simulink model "motor_model"  (R2022a)
settings: Solver=VariableStepAuto  StartTime=0.0  StopTime=T  FixedStep=0.001  RelTol=1e-3
values from neighbouring files (symbols this model uses):
  den_sys = sys.den{:}    [main.m]
  Kd = 10    [main.m]
  Ki = 100    [main.m]
  Kp = 300    [main.m]
  N = 80    [main.m]
  num_sys = sys.num{:}    [main.m]
undefined symbols (not defined in the file or in its folder): C_csd_den, C_csd_num, den_si, num_si
libraries: slpidlib x2, simulink x1
settings Model: Creator=michi  LastModifiedBy=michi

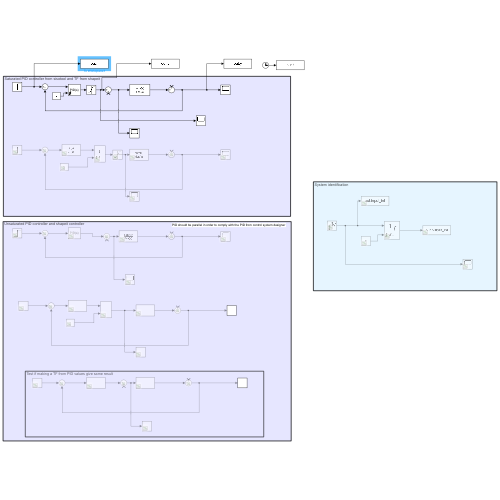
[thumbnail: Simulink's stored preview of the top-level diagram]
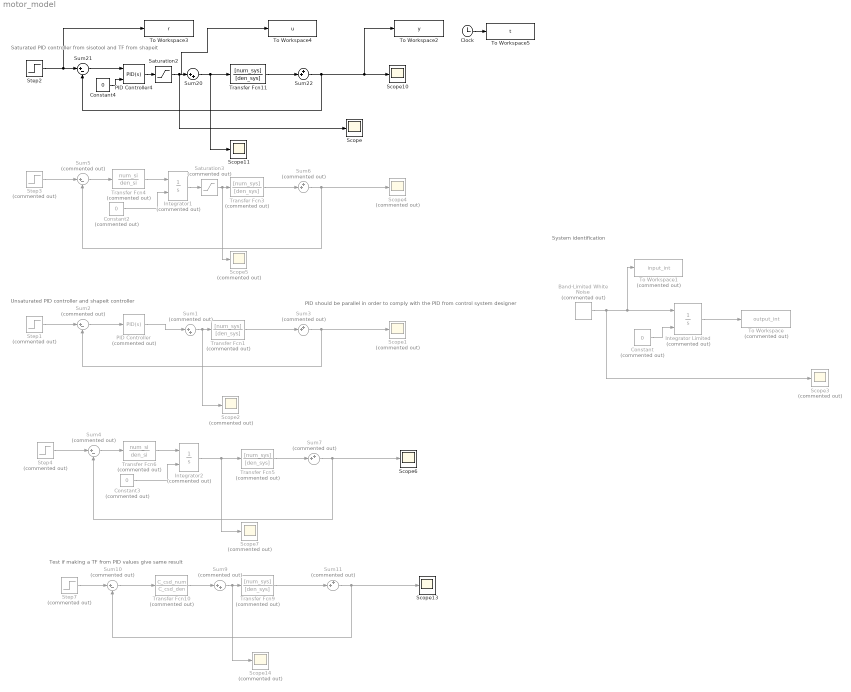
== system motor_model ==
  note: Test if making a TF from PID values give same result
  note: System identification
  note: PID should be parallel in order to comply with the PID from control system designer
  note: Unsaturated PID controller and shapeit controller
  note: Saturated PID controller from sisotool and TF from shapeit
  Band-Limited White Noise : simulink/Sources/Band-Limited White Noise  Commented=on  Cov=[1]  Ts=0.001  seed=[23341]
  Clock : Clock
  Constant : Constant  Commented=on  Value=0
  Constant2 : Constant  Commented=on  Value=0
  Constant3 : Constant  Commented=on  Value=0
  Constant4 : Constant  Value=0
  Integrator Limited : Integrator  Commented=on  ExternalReset=rising  LimitOutput=on  UpperSaturationLimit=3  LowerSaturationLimit=-3
  Integrator1 : Integrator  Commented=on  ExternalReset=rising  UpperSaturationLimit=3  LowerSaturationLimit=-3
  Integrator2 : Integrator  Commented=on  ExternalReset=rising  UpperSaturationLimit=3  LowerSaturationLimit=-3
  PID Controller : slpidlib/PID Controller  Commented=on  Controller=PID  Form=Parallel  TimeDomain=Continuous-time  UseExternalTs=off  SampleTime=-1  IntegratorMethod=Forward Euler  FilterMethod=Forward Euler  ControllerParametersSource=internal  P=Kp  I=Ki  UseKiTs=off  D=Kd  N=N  UseFilter=on  TunerSelectOption=Transfer Function Based (PID Tuner App)  InitialConditionSource=internal  InitialConditionForIntegrator=0  InitialConditionForFilter=0  DifferentiatorICPrevScaledInput=0  ExternalReset=none  TrackingMode=off  Kt=1  LimitOutput=off  SatLimitsSource=internal  UpperSaturationLimit=inf  LowerSaturationLimit=-inf  LinearizeAsGain=on  AntiWindupMode=none  Kb=1  POutMin=[]  POutMax=[]  IOutMin=[]  IOutMax=[]  DOutMin=[]  DOutMax=[]  NOutMin=[]  NOutMax=[]  SumOutMin=[]  SumOutMax=[]  SaturationOutMin=[]  SaturationOutMax=[]  PParamMin=[]  PParamMax=[]  IParamMin=[]  IParamMax=[]  DParamMin=[]  DParamMax=[]  NParamMin=[]  NParamMax=[]  KbParamMin=[]  KbParamMax=[]  KtParamMin=[]  KtParamMax=[]  KbOutMin=[]  KbOutMax=[]  KtOutMin=[]  KtOutMax=[]  IntegratorOutMin=[]  IntegratorOutMax=[]  FilterOutMin=[]  FilterOutMax=[]  SumI1OutMin=[]  SumI1OutMax=[]  SumI2OutMin=[]  SumI2OutMax=[]  SumI3OutMin=[]  SumI3OutMax=[]  SumI4OutMin=[]  SumI4OutMax=[]  SumDOutMin=[]  SumDOutMax=[]  DifferentiatorOutMin=[]  DifferentiatorOutMax=[]  FilterDiffOutCoefMin=[]  FilterDiffOutCoefMax=[]  ReciprocalOutMin=[]  ReciprocalOutMax=[]  SumDenOutMin=[]  SumDenOutMax=[]  SumNumOutMin=[]  SumNumOutMax=[]  DivideOutMin=[]  DivideOutMax=[]  UdiffTsProdOutMin=[]  UdiffTsProdOutMax=[]  NTsProdOutMin=[]  NTsProdOutMax=[]  UintegralTsProdOutMin=[]  UintegralTsProdOutMax=[]  UngainTsProdOutMin=[]  UngainTsProdOutMax=[]  IntegratorContinuousStateAttributes=''  IntegratorStateMustResolveToSignalObject=off  IntegratorRTWStateStorageClass=Auto  FilterContinuousStateAttributes=''  FilterStateMustResolveToSignalObject=off  FilterRTWStateStorageClass=Auto  ParallelPVariant=InternalParameters  IdealPVariant=Disabled  IVariant=InternalParameters  DVariant=InternalParameters  IntegratorVariant=Continuous  SatVariant=Disabled  AWVariant=Passthrough  PCopyVariant=Disabled  TRVariant=Disabled  FdbkBlocksVariant=Forward  IdealPFdbkVariant=Disabled  SatFdbkVariant=Disabled  DerivativeFilterVariant=ContFilter  NVariant=InternalParameters  NCopyVariant=Disabled  FilterICVariant=InternalICsFilter  IntegratorICVariant=InternalICs  ExternalResetVariant=Disabled  TRSumVariant=Passthrough  SumFdbkVariant=Disabled  SumVariant=Sum_PID  TsampFilterVariant=InternalTs  TsampNgainVariant=Passthrough  TsampIntegralVariant=Passthrough  ExternalSaturationOutDataTypeStr=Inherit: Same as second input  aMode=0
  PID Controller4 : slpidlib/PID Controller  Controller=PID  Form=Parallel  TimeDomain=Continuous-time  UseExternalTs=off  SampleTime=-1  IntegratorMethod=Forward Euler  FilterMethod=Forward Euler  ControllerParametersSource=internal  P=Kp  I=Ki  UseKiTs=off  D=Kd  N=N  UseFilter=on  TunerSelectOption=Transfer Function Based (PID Tuner App)  InitialConditionSource=internal  InitialConditionForIntegrator=0  InitialConditionForFilter=0  DifferentiatorICPrevScaledInput=0  ExternalReset=rising  TrackingMode=off  Kt=1  LimitOutput=off  SatLimitsSource=internal  UpperSaturationLimit=inf  LowerSaturationLimit=-inf  LinearizeAsGain=on  AntiWindupMode=none  Kb=1  POutMin=[]  POutMax=[]  IOutMin=[]  IOutMax=[]  DOutMin=[]  DOutMax=[]  NOutMin=[]  NOutMax=[]  SumOutMin=[]  SumOutMax=[]  SaturationOutMin=[]  SaturationOutMax=[]  PParamMin=[]  PParamMax=[]  IParamMin=[]  IParamMax=[]  DParamMin=[]  DParamMax=[]  NParamMin=[]  NParamMax=[]  KbParamMin=[]  KbParamMax=[]  KtParamMin=[]  KtParamMax=[]  KbOutMin=[]  KbOutMax=[]  KtOutMin=[]  KtOutMax=[]  IntegratorOutMin=[]  IntegratorOutMax=[]  FilterOutMin=[]  FilterOutMax=[]  SumI1OutMin=[]  SumI1OutMax=[]  SumI2OutMin=[]  SumI2OutMax=[]  SumI3OutMin=[]  SumI3OutMax=[]  SumI4OutMin=[]  SumI4OutMax=[]  SumDOutMin=[]  SumDOutMax=[]  DifferentiatorOutMin=[]  DifferentiatorOutMax=[]  FilterDiffOutCoefMin=[]  FilterDiffOutCoefMax=[]  ReciprocalOutMin=[]  ReciprocalOutMax=[]  SumDenOutMin=[]  SumDenOutMax=[]  SumNumOutMin=[]  SumNumOutMax=[]  DivideOutMin=[]  DivideOutMax=[]  UdiffTsProdOutMin=[]  UdiffTsProdOutMax=[]  NTsProdOutMin=[]  NTsProdOutMax=[]  UintegralTsProdOutMin=[]  UintegralTsProdOutMax=[]  UngainTsProdOutMin=[]  UngainTsProdOutMax=[]  IntegratorContinuousStateAttributes=''  IntegratorStateMustResolveToSignalObject=off  IntegratorRTWStateStorageClass=Auto  FilterContinuousStateAttributes=''  FilterStateMustResolveToSignalObject=off  FilterRTWStateStorageClass=Auto  ParallelPVariant=InternalParameters  IdealPVariant=Disabled  IVariant=InternalParameters  DVariant=InternalParameters  IntegratorVariant=Continuous  SatVariant=Disabled  AWVariant=Passthrough  PCopyVariant=Disabled  TRVariant=Disabled  FdbkBlocksVariant=Forward  IdealPFdbkVariant=Disabled  SatFdbkVariant=Disabled  DerivativeFilterVariant=ContFilter  NVariant=InternalParameters  NCopyVariant=Disabled  FilterICVariant=InternalICsFilter  IntegratorICVariant=InternalICs  ExternalResetVariant=ExternalReset  TRSumVariant=Passthrough  SumFdbkVariant=Disabled  SumVariant=Sum_PID  TsampFilterVariant=InternalTs  TsampNgainVariant=Passthrough  TsampIntegralVariant=Passthrough  ExternalSaturationOutDataTypeStr=Inherit: Same as second input  aMode=0
  Saturation2 : Saturate  UpperLimit=3  LowerLimit=-3
  Saturation3 : Saturate  Commented=on  UpperLimit=3  LowerLimit=-3
  Scope{,6,10..11,13} (5 alike) : Scope
  Scope{1..5,7,14} (7 alike) : Scope  Commented=on
  Step{1,3..4,7} (4 alike) : Step  Commented=on  After=0.01  SampleTime=0
  Step2 : Step  Before=-0.02  After=0.02  SampleTime=0
  Sum1 : Sum  Commented=on  Inputs=|++
  Sum{2,4..5,10} (4 alike) : Sum  Commented=on  Inputs=|+-
  Sum{3,6..7,11} (4 alike) : Sum  Commented=on  Inputs=++|
  Sum20 : Sum  Inputs=|++
  Sum21 : Sum  Inputs=|+-
  Sum22 : Sum  Inputs=++|
  Sum9 : Sum  Commented=on  Inputs=|++
  To Workspace : ToWorkspace  Commented=on  VariableName=output_int  SampleTime=-1
  To Workspace1 : ToWorkspace  Commented=on  VariableName=input_int  SampleTime=-1
  To Workspace2 : ToWorkspace  VariableName=y  SampleTime=-1
  To Workspace3 : ToWorkspace  VariableName=r  SampleTime=-1
  To Workspace4 : ToWorkspace  VariableName=u  SampleTime=-1
  To Workspace5 : ToWorkspace  VariableName=t  SampleTime=-1
  Transfer Fcn{1,3,5,9} (4 alike) : TransferFcn  Commented=on  Numerator=[num_sys]  Denominator=[den_sys]
  Transfer Fcn10 : TransferFcn  Commented=on  Numerator=C_csd_num  Denominator=C_csd_den
  Transfer Fcn11 : TransferFcn  Numerator=[num_sys]  Denominator=[den_sys]
  Transfer Fcn4 : TransferFcn  Commented=on  Numerator=num_si  Denominator=den_si
  Transfer Fcn6 : TransferFcn  Commented=on  Numerator=num_si  Denominator=den_si
  wires:
  Constant/1 -> Integrator Limited/2
  Band-Limited White Noise/1 -> Scope3/1, To Workspace1/1, Integrator Limited/1
  Integrator Limited/1 -> To Workspace/1
  PID Controller4/1 -> Saturation2/1
  Sum21/1 -> PID Controller4/1
  Sum20/1 -> Transfer Fcn11/1, Scope11/1
  Constant4/1 -> PID Controller4/2
  Step2/1 -> To Workspace3/1, Sum21/1
  Saturation2/1 -> Scope/1, To Workspace4/1, Sum20/1
  Sum22/1 -> To Workspace2/1, Scope10/1, Sum21/2
  Sum3/1 -> Scope1/1, Sum2/2
  Transfer Fcn1/1 -> Sum3/2
  Step1/1 -> Sum2/1
  Sum1/1 -> Scope2/1, Transfer Fcn1/1
  Step3/1 -> Sum5/1
  Sum6/1 -> Scope4/1, Sum5/2
  Transfer Fcn3/1 -> Sum6/2
  Transfer Fcn4/1 -> Integrator1/1
  Sum5/1 -> Transfer Fcn4/1
  Sum4/1 -> Transfer Fcn6/1
  Transfer Fcn6/1 -> Integrator2/1
  Step4/1 -> Sum4/1
  Transfer Fcn5/1 -> Sum7/2
  Integrator2/1 -> Scope7/1, Transfer Fcn5/1
  Sum7/1 -> Scope6/1, Sum4/2
  Constant2/1 -> Integrator1/2
  Constant3/1 -> Integrator2/2
  Integrator1/1 -> Saturation3/1
  Saturation3/1 -> Scope5/1, Transfer Fcn3/1
  Step7/1 -> Sum10/1
  Transfer Fcn9/1 -> Sum11/2
  Sum9/1 -> Scope14/1, Transfer Fcn9/1
  Sum11/1 -> Scope13/1, Sum10/2
  Sum10/1 -> Transfer Fcn10/1
  Transfer Fcn10/1 -> Sum9/1
  Sum2/1 -> PID Controller/1
  PID Controller/1 -> Sum1/1
  Clock/1 -> To Workspace5/1
  Transfer Fcn11/1 -> Sum22/2
